simulink model "prob5_drag"  (R2026a)
settings: Solver=ode45  StopTime=5
settings Model: Creator=tdxt  LastModifiedBy=tdxt

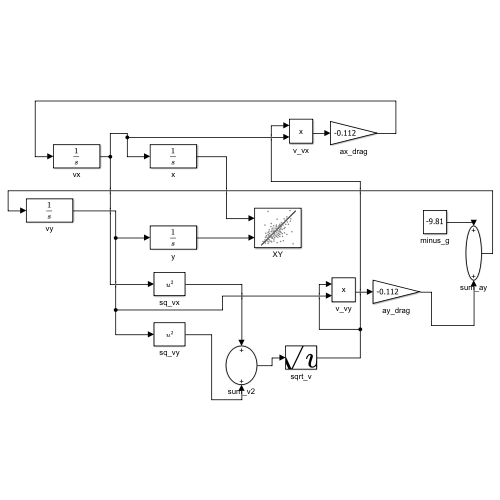
[thumbnail: Simulink's stored preview of the top-level diagram]
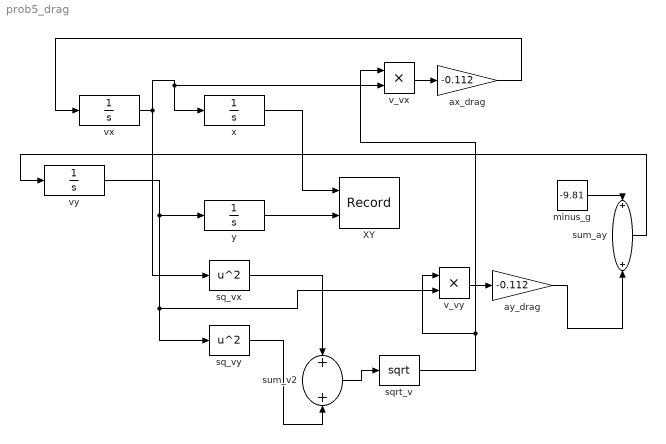
== system prob5_drag ==
  XY : Record  NumPorts=2.0  FileSettingsInternal="{\"entries\":[{\"content\":{\"excelSettings\":{\"content\":{},\"type\":\"Streamout.ExcelSettings\"},\"parquetSettings\":{\"content\":{},\"type\":\"Streamout.ParquetSettings\"}},\"type\":\"Streamout.FileSettingStorage\",\"uuid\":\"\"}],\"packageUris\":[\"http:\\/\\/schema.mathworks.com\\/mf0\\/streamout_blocks\\/R2020a\"],\"version\":\"1.0\"}"  FrameSettings=[0, 0]  Layout=[1 1]  SignalsInternal="{\"entries\":[{\"content\":{\"signals\":[{\"content\":{\"blockPath\":[],\"dimensions\":[1],\"domain\":\"\",\"lineColor\":\"#a2142f\",\"plots\":[ 1 ],\"port\":1,\"sid\":[\"\"],\"signalID\":1,\"signalName\":\"x\"},\"type\":\"RecordBlkView.Signal\",\"uuid\":\"\"},{\"content\":{\"blockPath\":[],\"dimensions\":[1],\"domain\":\"\",\"lineColor\":\"#139fff\",\"plots\":[ 1 ],\"port\":2,\"sid\":[\"\"],\"signalID\":2,\"signalName\":\"y\"},\"type\":\"RecordBlkView.Signal\",\"uuid\":\"\"}]},\"type\":\"RecordBlkView.InputSignals\",\"uuid\":\"\"}],\"packageUris\":[\"http:\\/\\/schema.mathworks.com\\/mf0\\/streamout_blocks\\/R2020a\"],\"version\":\"1.0\"}"  VisualizationBindings="{\"xyplotplugin\":{\"info\":[{\"series\":[{\"bindingParametersList\":[{\"parameter\":\"X-Axis\",\"signalID\":1,\"signalName\":\"x\"},{\"parameter\":\"Y-Axis\",\"signalID\":2,\"signalName\":\"y\"}],\"seriesID\":0}],\"subplotID\":1}]}}"  CompatibilityTag=XY
  ax_drag : Gain  Gain=-0.112
  ay_drag : Gain  Gain=-0.112
  minus_g : Constant  Value=-9.81
  sq_vx : Math  Operator=square
  sq_vy : Math  Operator=square
  sqrt_v : Math  Operator=sqrt
  sum_ay : Sum
  sum_v2 : Sum
  v_vx : Product
  v_vy : Product
  vx : Integrator  InitialCondition=17.9981
  vy : Integrator  InitialCondition=21.4492
  x : Integrator
  y : Integrator
  wires:
  sq_vx/1 -> sum_v2/1
  vx/1 -> v_vx/2, x/1, sq_vx/1
  vy/1 -> sq_vy/1, v_vy/2, y/1
  x/1 -> XY/1
  y/1 -> XY/2
  sqrt_v/1 -> v_vy/1, v_vx/1
  sq_vy/1 -> sum_v2/2
  sum_v2/1 -> sqrt_v/1
  v_vx/1 -> ax_drag/1
  v_vy/1 -> ay_drag/1
  ax_drag/1 -> vx/1
  ay_drag/1 -> sum_ay/2
  minus_g/1 -> sum_ay/1
  sum_ay/1 -> vy/1
